simulink model "assignment_part_1_simulink"  (R2025b)
settings: Solver=FixedStepAuto  StartTime=0.0  StopTime=20  FixedStep=0.0001  RelTol=1e-3
values from neighbouring files (symbols this model uses):
  VT = 0.72      + 0.0667 .* x      + 0.0885 .* x .* (x - 1.2)      - 0.0381 .* x .* (x - 1.2) .* (x - 3.2)      + 0.0068 .* x .* (x - 1.2) .* (x - 3.2) .* (x - 6)      - 0.0011 .* x .* (x - 1.2) .* (x - 3.2) .* (x - 6) .* (x - 9)    [VT_of_t.m]
undefined symbols (not defined in the file or in its folder): BS, Gc, JM, JW, KC, KD, KE, KH, KS, KT, KV, KY, L, R, RM, RW, VD
settings Model: Creator=m4z3o  LastModifiedBy=m4z3o

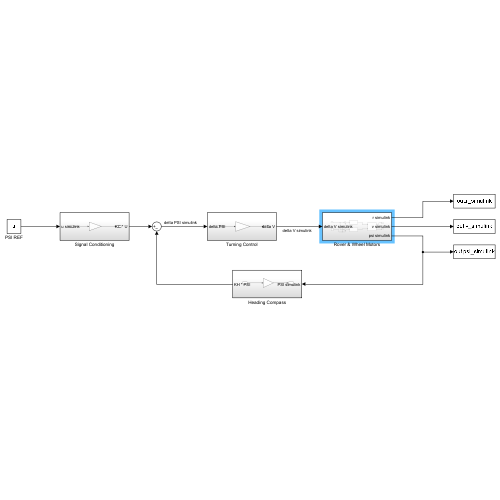
[thumbnail: Simulink's stored preview of the top-level diagram]
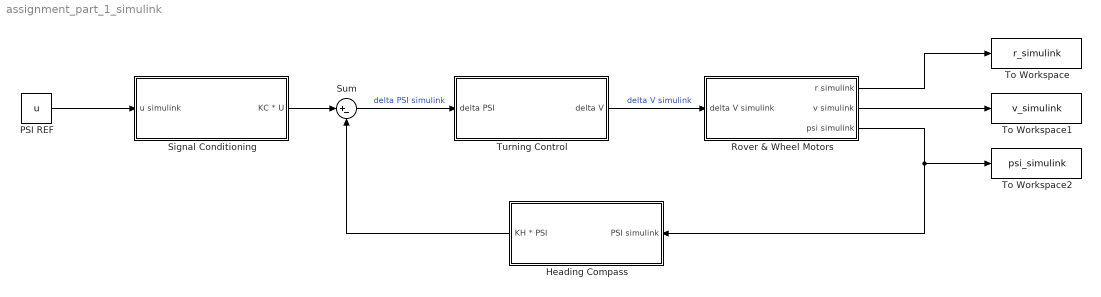
== system assignment_part_1_simulink ==
  Heading Compass : Subsystem
  PSI REF : Constant  Value=u
  Rover & Wheel Motors : Subsystem
  Signal Conditioning : Subsystem
  Sum : Sum  Inputs=|+-
  To Workspace : ToWorkspace  VariableName=r_simulink  SaveFormat=Timeseries  SampleTime=-1
  To Workspace1 : ToWorkspace  VariableName=v_simulink  SaveFormat=Timeseries  SampleTime=-1
  To Workspace2 : ToWorkspace  VariableName=psi_simulink  SaveFormat=Timeseries  SampleTime=-1
  Turning Control : Subsystem
  wires:
  PSI REF/1 -> Signal Conditioning/1(u simulink)
  Signal Conditioning/1(KC * U) -> Sum/1
  Sum/1 -> Turning Control/1(delta PSI)  "delta PSI simulink"
  Turning Control/1(delta V) -> Rover & Wheel Motors/1(delta V simulink)  "delta V simulink"
  Heading Compass/1("KH * PSI ") -> Sum/2
  Rover & Wheel Motors/1(r simulink) -> To Workspace/1
  Rover & Wheel Motors/3(psi simulink) -> Heading Compass/1(PSI simulink), To Workspace2/1
  Rover & Wheel Motors/2(v simulink) -> To Workspace1/1

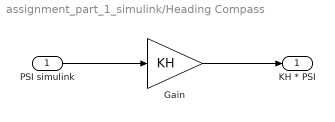
== system assignment_part_1_simulink/Heading Compass ==
  PSI simulink : Inport
  Gain : Gain  Gain=KH
  "KH * PSI " : Outport
  wires:
  PSI simulink/1 -> Gain/1
  Gain/1 -> "KH * PSI "/1

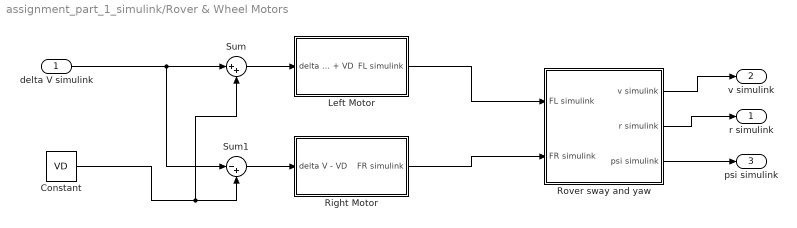
== system assignment_part_1_simulink/Rover & Wheel Motors ==
  delta V simulink : Inport
  Constant : Constant  Value=VD
  Left Motor : Subsystem
  Right Motor : Subsystem
  Rover sway and yaw : Subsystem
  Sum : Sum  Inputs=|++
  Sum1 : Sum  Inputs=|-+
  r simulink : Outport
  v simulink : Outport  Port=2
  psi simulink : Outport  Port=3
  wires:
  Rover sway and yaw/1(v simulink) -> v simulink/1
  Rover sway and yaw/2(r simulink) -> r simulink/1
  Rover sway and yaw/3(psi simulink) -> psi simulink/1
  Constant/1 -> Sum/2, Sum1/2
  Sum1/1 -> Right Motor/1(delta V - VD)
  Sum/1 -> Left Motor/1(delta V + VD)
  delta V simulink/1 -> Sum1/1, Sum/1
  Left Motor/1(FL simulink) -> Rover sway and yaw/1(FL simulink)
  Right Motor/1(FR simulink) -> Rover sway and yaw/2(FR simulink)

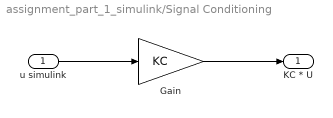
== system assignment_part_1_simulink/Signal Conditioning ==
  u simulink : Inport
  Gain : Gain  Gain=KC
  KC * U : Outport
  wires:
  u simulink/1 -> Gain/1
  Gain/1 -> KC * U/1

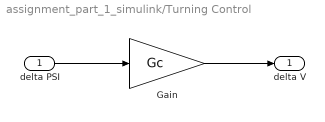
== system assignment_part_1_simulink/Turning Control ==
  delta PSI : Inport
  Gain : Gain  Gain=Gc
  delta V : Outport
  wires:
  delta PSI/1 -> Gain/1
  Gain/1 -> delta V/1

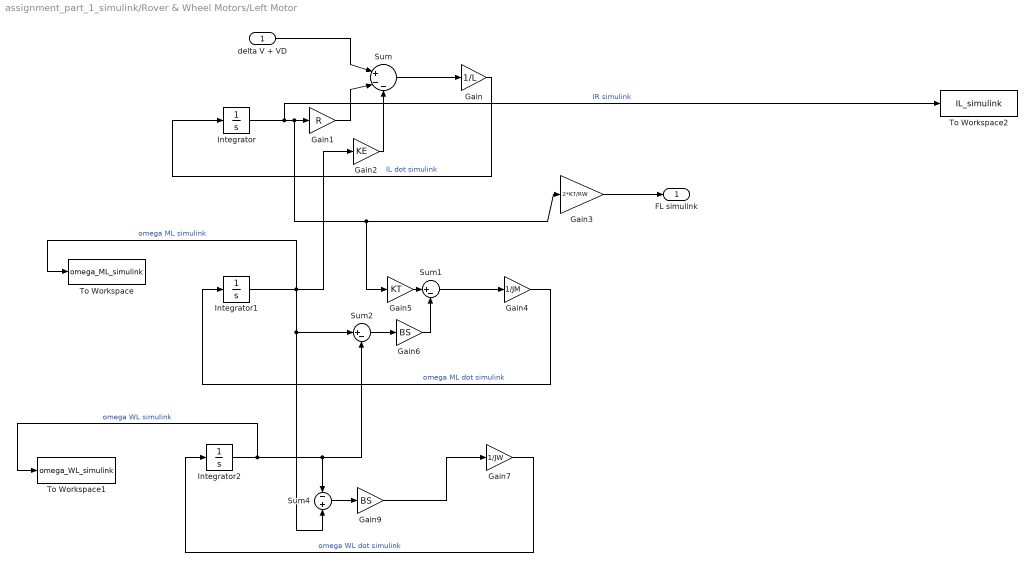
== system assignment_part_1_simulink/Rover & Wheel Motors/Left Motor ==
  delta V + VD : Inport
  Gain : Gain  Gain=1/L
  Gain1 : Gain  Gain=R
  Gain2 : Gain  Gain=KE
  Gain3 : Gain  Gain=2*KT/RW
  Gain4 : Gain  Gain=1/JM
  Gain5 : Gain  Gain=KT
  Gain6 : Gain  Gain=BS
  Gain7 : Gain  Gain=1/JW
  Gain9 : Gain  Gain=BS
  Integrator : Integrator
  Integrator1 : Integrator
  Integrator2 : Integrator
  Sum : Sum  Inputs=|+--
  Sum1 : Sum  Inputs=|+-
  Sum2 : Sum  Inputs=|+-
  Sum4 : Sum  Inputs=-+
  To Workspace : ToWorkspace  VariableName=omega_ML_simulink  SaveFormat=Timeseries  SampleTime=-1
  To Workspace1 : ToWorkspace  VariableName=omega_WL_simulink  SaveFormat=Timeseries  SampleTime=-1
  To Workspace2 : ToWorkspace  VariableName=IL_simulink  SaveFormat=Timeseries  SampleTime=-1
  FL simulink : Outport
  wires:
  delta V + VD/1 -> Sum/1
  Gain1/1 -> Sum/2
  Gain/1 -> Integrator/1  "IL dot simulink"
  Sum/1 -> Gain/1
  Integrator1/1 -> To Workspace/1, Sum4/2, Sum2/1, Gain2/1  "omega ML simulink"
  Gain2/1 -> Sum/3
  Gain3/1 -> FL simulink/1
  Sum1/1 -> Gain4/1
  Gain4/1 -> Integrator1/1  "omega ML dot simulink"
  Gain5/1 -> Sum1/1
  Gain6/1 -> Sum1/2
  Sum2/1 -> Gain6/1
  Gain7/1 -> Integrator2/1  "omega WL dot simulink"
  Sum4/1 -> Gain9/1
  Gain9/1 -> Gain7/1
  Integrator2/1 -> To Workspace1/1, Sum2/2, Sum4/1  "omega WL simulink"
  Integrator/1 -> To Workspace2/1, Gain3/1, Gain5/1, Gain1/1  "IR simulink"

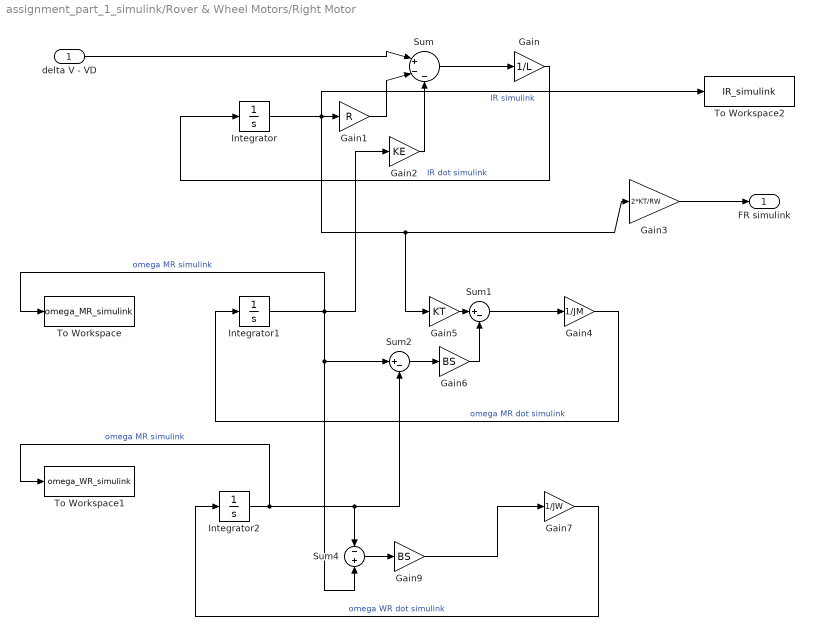
== system assignment_part_1_simulink/Rover & Wheel Motors/Right Motor ==
  delta V - VD : Inport
  Gain : Gain  Gain=1/L
  Gain1 : Gain  Gain=R
  Gain2 : Gain  Gain=KE
  Gain3 : Gain  Gain=2*KT/RW
  Gain4 : Gain  Gain=1/JM
  Gain5 : Gain  Gain=KT
  Gain6 : Gain  Gain=BS
  Gain7 : Gain  Gain=1/JW
  Gain9 : Gain  Gain=BS
  Integrator : Integrator
  Integrator1 : Integrator
  Integrator2 : Integrator
  Sum : Sum  Inputs=|+--
  Sum1 : Sum  Inputs=|+-
  Sum2 : Sum  Inputs=|+-
  Sum4 : Sum  Inputs=-+
  To Workspace : ToWorkspace  VariableName=omega_MR_simulink  SaveFormat=Timeseries  SampleTime=-1
  To Workspace1 : ToWorkspace  VariableName=omega_WR_simulink  SaveFormat=Timeseries  SampleTime=-1
  To Workspace2 : ToWorkspace  VariableName=IR_simulink  SaveFormat=Timeseries  SampleTime=-1
  FR simulink : Outport
  wires:
  delta V - VD/1 -> Sum/1
  Gain1/1 -> Sum/2
  Gain/1 -> Integrator/1  "IR dot simulink"
  Sum/1 -> Gain/1
  Gain2/1 -> Sum/3
  Gain3/1 -> FR simulink/1
  Sum1/1 -> Gain4/1
  Gain4/1 -> Integrator1/1  "omega MR dot simulink"
  Gain5/1 -> Sum1/1
  Gain6/1 -> Sum1/2
  Sum2/1 -> Gain6/1
  Gain7/1 -> Integrator2/1  "omega WR dot simulink"
  Integrator/1 -> To Workspace2/1, Gain3/1, Gain5/1, Gain1/1  "IR simulink"
  Sum4/1 -> Gain9/1
  Gain9/1 -> Gain7/1
  Integrator1/1 -> To Workspace/1, Sum4/2, Sum2/1, Gain2/1  "omega MR simulink"
  Integrator2/1 -> To Workspace1/1, Sum2/2, Sum4/1  "omega MR simulink"

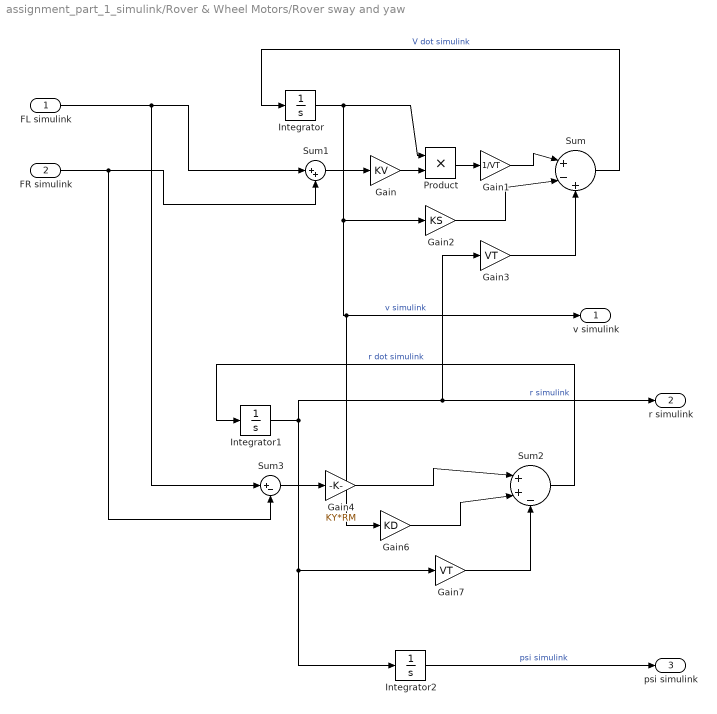
== system assignment_part_1_simulink/Rover & Wheel Motors/Rover sway and yaw ==
  FL simulink : Inport
  FR simulink : Inport  Port=2
  Gain : Gain  Gain=KV
  Gain1 : Gain  Gain=1/VT
  Gain2 : Gain  Gain=KS
  Gain3 : Gain  Gain=VT
  Gain4 : Gain  Gain=KY*RM
  Gain6 : Gain  Gain=KD
  Gain7 : Gain  Gain=VT
  Integrator : Integrator
  Integrator1 : Integrator  InitialCondition=1
  Integrator2 : Integrator  InitialCondition=-12*pi/180
  Product : Product
  Sum : Sum  Inputs=|+-+
  Sum1 : Sum  Inputs=|++
  Sum2 : Sum  Inputs=|++-
  Sum3 : Sum  Inputs=|+-
  v simulink : Outport
  r simulink : Outport  Port=2
  psi simulink : Outport  Port=3
  wires:
  Sum/1 -> Integrator/1  "V dot simulink"
  Integrator/1 -> Gain2/1, Gain6/1, v simulink/1, Product/1  "v simulink"
  Sum1/1 -> Gain/1
  Gain/1 -> Product/2
  Product/1 -> Gain1/1
  Gain1/1 -> Sum/1
  Gain2/1 -> Sum/2
  Gain3/1 -> Sum/3
  Integrator1/1 -> Gain7/1, Integrator2/1, Gain3/1, r simulink/1  "r simulink"
  Sum3/1 -> Gain4/1
  FR simulink/1 -> Sum3/2, Sum1/2
  FL simulink/1 -> Sum3/1, Sum1/1
  Gain7/1 -> Sum2/3
  Gain4/1 -> Sum2/1
  Sum2/1 -> Integrator1/1  "r dot simulink"
  Gain6/1 -> Sum2/2
  Integrator2/1 -> psi simulink/1  "psi simulink"
